simulink model "blockdemo"  (Simulink 6.3)
settings: Solver=ode45  StartTime=0.0  StopTime=100  RelTol=1e-3
InitFcn:
  | %% DSPBuilder Start
  | alt_dspbuilder_update_model(bdroot)
  | %% DSPBuilder End
libraries: allblocks_alteradspbuilder2 x7
settings Model: Creator=cpurcell  LastModifiedBy=delphick
settings OptimizationCC: BlockReduction=off  BooleanDataType=off  InlineInvariantSignals=on
settings DebuggingCC: SolverPrmCheckMsg=none
settings HardwareCC: TargetUnknown=on

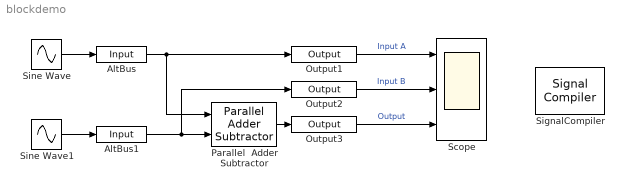
== system blockdemo ==
  AltBus : allblocks_alteradspbuilder2/Input  iofile=C:\workspace_clean\Documentation\DesignExamples\Tutorials\UnitBlocks\Arithmetic\ParallelAdder\tb_blockdemo\blockdemo_AltBus.salt  BusType=Signed Integer  bwl=5  bwr=4  SpecifyClock=off  PORTTYPE=Input
  AltBus1 : allblocks_alteradspbuilder2/Input  iofile=C:\workspace_clean\Documentation\DesignExamples\Tutorials\UnitBlocks\Arithmetic\ParallelAdder\tb_blockdemo\blockdemo_AltBus1.salt  BusType=Signed Integer  bwl=5  bwr=4  SpecifyClock=off  PORTTYPE=Input
  Output1 : allblocks_alteradspbuilder2/Output  iofile=C:\workspace_clean\Documentation\DesignExamples\Tutorials\UnitBlocks\Arithmetic\ParallelAdder\tb_blockdemo\blockdemo_Output1.capture  BusType=Signed Integer  bwl=5  bwr=0  PORTTYPE=Output
  Output2 : allblocks_alteradspbuilder2/Output  iofile=C:\workspace_clean\Documentation\DesignExamples\Tutorials\UnitBlocks\Arithmetic\ParallelAdder\tb_blockdemo\blockdemo_Output2.capture  BusType=Signed Integer  bwl=5  bwr=0  PORTTYPE=Output
  Output3 : allblocks_alteradspbuilder2/Output  iofile=C:\workspace_clean\Documentation\DesignExamples\Tutorials\UnitBlocks\Arithmetic\ParallelAdder\tb_blockdemo\blockdemo_Output3.capture  BusType=Signed Integer  bwl=5  bwr=0  PORTTYPE=Output
  Parallel  Adder Subtractor : allblocks_alteradspbuilder2/Parallel Adder Subtractor  number_of_inputs=2  direction=+++  use_pipeline=off  phase_selection=1  use_ena=off  use_aclr=off
  Scope : Scope  NumInputPorts=3
      settings: YMin=-20~-20~-2  YMax=20~20~1
  SignalCompiler : allblocks_alteradspbuilder2/Signal Compiler  DeviceFamily=Stratix IV  DeviceName=AUTO  EnableSignalTap=off  SignalTapDepth=128  UseBoardBlock=off  StpUseDefaultClock=on  StpClock=clock
  Sine Wave : Sin  Amplitude=15  Frequency=0.1  Phase=pi  SampleTime=0
  Sine Wave1 : Sin  Amplitude=15  Frequency=0.1  SampleTime=0
  wires:
  AltBus/1 -> Parallel  Adder Subtractor/1, Output1/1
  Sine Wave/1 -> AltBus/1
  Parallel  Adder Subtractor/1 -> Output3/1
  AltBus1/1 -> Parallel  Adder Subtractor/2, Output2/1
  Sine Wave1/1 -> AltBus1/1
  Output1/1 -> Scope/1  "Input A"
  Output2/1 -> Scope/2  "Input B"
  Output3/1 -> Scope/3  "Output"
